simulink model "progetto_sim_controllato"  (R2025b)
settings: Solver=VariableStepAuto  StartTime=0.0  StopTime=1e3  RelTol=1e-3
values from neighbouring files (symbols this model uses):
  d0 = [110 130 100 160]    [backup_id_macchine.mat]    (also in id_macchine.mat)
  dmin = 4    [backup_id_macchine.mat]    (also in id_macchine.mat)
  mDist = [156.727602966 155.419177889 157.307233343 156.111472907]    [backup_id_macchine.mat]    (also in id_macchine.mat = [156.911734511 155.758692096 157.721037406 156.538222818])
  t_cth = 3    [backup_id_macchine.mat]    (also in id_macchine.mat)
  Ts = 2    [backup_id_macchine.mat]    (also in id_macchine.mat)
  umax = 600    [backup_id_macchine.mat]    (also in id_macchine.mat)
  umin = -600    [backup_id_macchine.mat]    (also in id_macchine.mat)
  v0 = [10 12 15 9 10]    [backup_id_macchine.mat]    (also in id_macchine.mat)
  vMedio = [9.99088198605 9.9851530035 9.98261849858 9.98180014012]    [backup_id_macchine.mat]    (also in id_macchine.mat = [10.0026522625 10.0031571294 10.0027874656 10.0025052689])
  x0 = [10 12 15 9 10]    [backup_id_macchine.mat]    (also in id_macchine.mat)
undefined symbols (not defined in the file or in its folder): s2totss, s3totss, s4totss, s5totss
libraries: mpclib x4
settings Model: Creator=david  LastModifiedBy=david

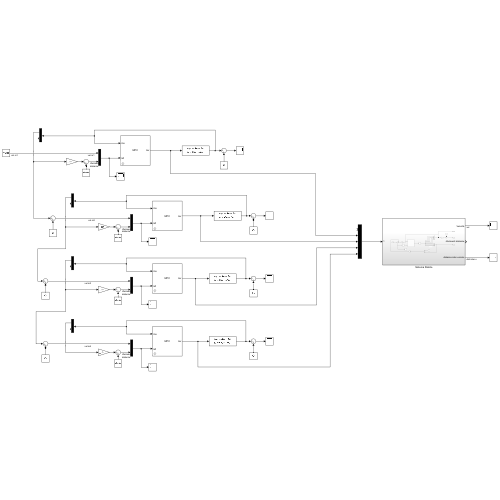
[thumbnail: Simulink's stored preview of the top-level diagram]
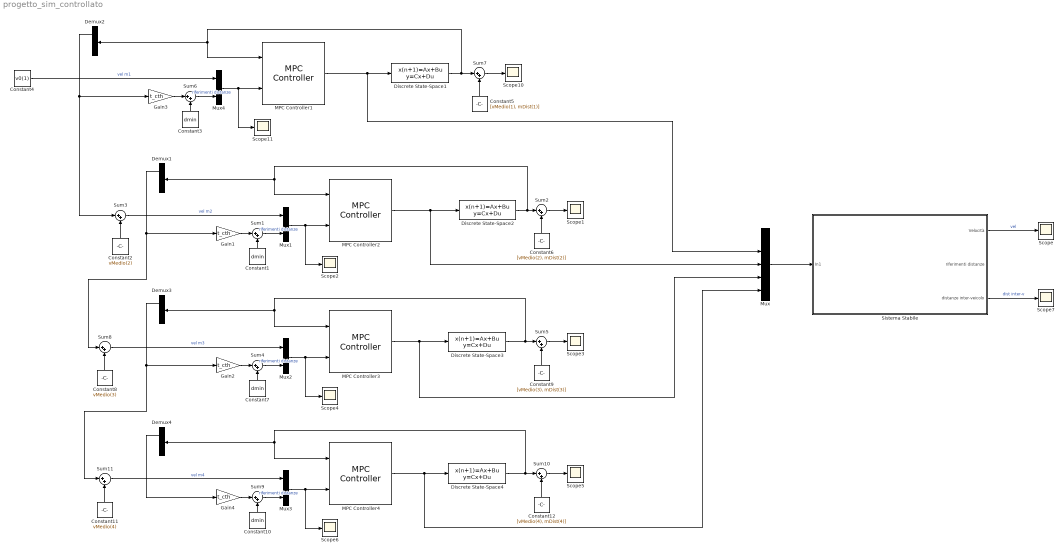
== system progetto_sim_controllato ==
  Constant{1,3,7,10} (4 alike) : Constant  Value=dmin
  Constant11 : Constant  Value=vMedio(4)
  Constant12 : Constant  Value=[vMedio(4), mDist(4)]
  Constant2 : Constant  Value=vMedio(2)
  Constant4 : Constant  Value=v0(1)
  Constant5 : Constant  Value=[vMedio(1), mDist(1)]
  Constant6 : Constant  Value=[vMedio(2), mDist(2)]
  Constant8 : Constant  Value=vMedio(3)
  Constant9 : Constant  Value=[vMedio(3), mDist(3)]
  Demux{1..4} (4 alike) : Demux  Outputs=2
  Discrete State-Space1 : DiscreteStateSpace  A=s2totss.A  B=s2totss.B  C=s2totss.C  D=s2totss.D  SampleTime=Ts
  Discrete State-Space2 : DiscreteStateSpace  A=s3totss.A  B=s3totss.B  C=s3totss.C  D=s3totss.D  SampleTime=Ts
  Discrete State-Space3 : DiscreteStateSpace  A=s4totss.A  B=s4totss.B  C=s4totss.C  D=s4totss.D  SampleTime=Ts
  Discrete State-Space4 : DiscreteStateSpace  A=s5totss.A  B=s5totss.B  C=s5totss.C  D=s5totss.D  SampleTime=Ts
  Gain{1..4} (4 alike) : Gain  Gain=t_cth
  MPC Controller1 : mpclib/MPC Controller  SCDEnableBlockLinearizationSpecification=on  mpcobj=mpcs2  is_multiple=0  enable_value=0  return_u0=off  updateMPCinCallerWorkspace=on  md_inport=off  mv_inport=off  uref_inport=off  return_cost=off  return_mvseq=off  return_qpstatus=off  return_xseq=off  return_state=off  return_ovseq=off  state_inport=off  umin_inport=off  umax_inport=off  ymin_inport=off  ymax_inport=off  cc_inport=off  ywt_inport=off  uwt_inport=off  duwt_inport=off  rhoeps_inport=off  pm_inport=off  MaximumP=10  HorizonChoice=FixedHorizon  n_ts=2  n_p=10  n_mv=1  n_md=0  n_ud=0  n_mo=2  n_uo=0  BlockDataType=double  SampleTimeInherited=off  switch_inport=off
  MPC Controller2 : mpclib/MPC Controller  SCDEnableBlockLinearizationSpecification=on  mpcobj=mpcs3  is_multiple=0  enable_value=0  return_u0=off  updateMPCinCallerWorkspace=on  md_inport=off  mv_inport=off  uref_inport=off  return_cost=off  return_mvseq=off  return_qpstatus=off  return_xseq=off  return_state=off  return_ovseq=off  state_inport=off  umin_inport=off  umax_inport=off  ymin_inport=off  ymax_inport=off  cc_inport=off  ywt_inport=off  uwt_inport=off  duwt_inport=off  rhoeps_inport=off  pm_inport=off  MaximumP=10  HorizonChoice=FixedHorizon  n_ts=2  n_p=10  n_mv=1  n_md=0  n_ud=0  n_mo=2  n_uo=0  BlockDataType=double  SampleTimeInherited=off  switch_inport=off
  MPC Controller3 : mpclib/MPC Controller  SCDEnableBlockLinearizationSpecification=on  mpcobj=mpcs4  is_multiple=0  enable_value=0  return_u0=off  updateMPCinCallerWorkspace=on  md_inport=off  mv_inport=off  uref_inport=off  return_cost=off  return_mvseq=off  return_qpstatus=off  return_xseq=off  return_state=off  return_ovseq=off  state_inport=off  umin_inport=off  umax_inport=off  ymin_inport=off  ymax_inport=off  cc_inport=off  ywt_inport=off  uwt_inport=off  duwt_inport=off  rhoeps_inport=off  pm_inport=off  MaximumP=10  HorizonChoice=FixedHorizon  n_ts=2  n_p=10  n_mv=1  n_md=0  n_ud=0  n_mo=2  n_uo=0  BlockDataType=double  SampleTimeInherited=off  switch_inport=off
  MPC Controller4 : mpclib/MPC Controller  SCDEnableBlockLinearizationSpecification=on  mpcobj=mpcs5  is_multiple=0  enable_value=0  return_u0=off  updateMPCinCallerWorkspace=on  md_inport=off  mv_inport=off  uref_inport=off  return_cost=off  return_mvseq=off  return_qpstatus=off  return_xseq=off  return_state=off  return_ovseq=off  state_inport=off  umin_inport=off  umax_inport=off  ymin_inport=off  ymax_inport=off  cc_inport=off  ywt_inport=off  uwt_inport=off  duwt_inport=off  rhoeps_inport=off  pm_inport=off  MaximumP=10  HorizonChoice=FixedHorizon  n_ts=2  n_p=10  n_mv=1  n_md=0  n_ud=0  n_mo=2  n_uo=0  BlockDataType=double  SampleTimeInherited=off  switch_inport=off
  Mux : Mux  Inputs=5
  Mux{1..4} (4 alike) : Mux  Inputs=2
  Scope{,1..7,10..11} (10 alike) : Scope
      Scope settings: ActiveDisplayYMinimum=7.1891776875022071  ActiveDisplayYMaximum=15.867869145833088  DataLoggingVariableName=ScopeData6
      Scope1 settings: ActiveDisplayYMinimum=10.60470416126369  ActiveDisplayYMaximum=10.628775186898299
      Scope10 settings: ActiveDisplayYMinimum=9.85178753278167  ActiveDisplayYMaximum=10.21313439515283  DataLoggingVariableName=ScopeData21
      Scope11 settings: ActiveDisplayYMinimum=-1  ActiveDisplayYMaximum=1  DataLoggingVariableName=ScopeData22
      Scope2 settings: ActiveDisplayYMinimum=9.99782194789179  ActiveDisplayYMaximum=10.03576388043639
      Scope3 settings: ActiveDisplayYMinimum=9.8157241607277683  ActiveDisplayYMaximum=12.871337364076957  DataLoggingVariableName=ScopeData2
      Scope4 settings: ActiveDisplayYMinimum=9.99782194789179  ActiveDisplayYMaximum=10.03576388043639  DataLoggingVariableName=ScopeData3
      Scope5 settings: ActiveDisplayYMinimum=5.3910159181870654  ActiveDisplayYMaximum=20.171430503682927  DataLoggingVariableName=ScopeData4
      Scope6 settings: ActiveDisplayYMinimum=1.7380163806894  ActiveDisplayYMaximum=24.357852573795405  DataLoggingVariableName=ScopeData5
      Scope7 settings: ActiveDisplayYMinimum=40.1130251052208  ActiveDisplayYMaximum=173.32077498830881  DataLoggingVariableName=ScopeData7
  Sistema Stabile : Subsystem
  Sum{1..11} (11 alike) : Sum  Inputs=|++
  wires:
  Constant5/1 -> Sum7/2
  Sum6/1 -> Mux4/2  "riferimenti distanze"
  Mux4/1 -> Scope11/1, MPC Controller1/2
  Sum7/1 -> Scope10/1
  Constant3/1 -> Sum6/2
  Gain3/1 -> Sum6/1
  MPC Controller1/1 -> Mux/2, Discrete State-Space1/1
  Discrete State-Space1/1 -> Sum7/1, MPC Controller1/1, Demux2/1
  Gain1/1 -> Sum1/1
  MPC Controller2/1 -> Mux/3, Discrete State-Space2/1
  Discrete State-Space2/1 -> MPC Controller2/1, Demux1/1, Sum2/1
  Sum1/1 -> Mux1/2  "riferimenti distanze"
  Mux1/1 -> Scope2/1, MPC Controller2/2
  Demux1/1 -> Sum8/1, Gain1/1
  Constant1/1 -> Sum1/2
  Sum2/1 -> Scope1/1
  Constant6/1 -> Sum2/2
  Sum3/1 -> Mux1/1  "vel m2"
  Constant2/1 -> Sum3/2
  Demux3/1 -> Sum11/1, Gain2/1
  Constant7/1 -> Sum4/2
  Sum5/1 -> Scope3/1
  Constant9/1 -> Sum5/2
  Mux2/1 -> Scope4/1, MPC Controller3/2
  Discrete State-Space3/1 -> Sum5/1, MPC Controller3/1, Demux3/1
  Gain2/1 -> Sum4/1
  MPC Controller3/1 -> Mux/4, Discrete State-Space3/1
  Sum4/1 -> Mux2/2  "riferimenti distanze"
  Constant8/1 -> Sum8/2
  Sum8/1 -> Mux2/1  "vel m3"
  Demux2/1 -> Sum3/1, Gain3/1
  Sum11/1 -> Mux3/1  "vel m4"
  Constant11/1 -> Sum11/2
  Sum9/1 -> Mux3/2  "riferimenti distanze"
  MPC Controller4/1 -> Mux/5, Discrete State-Space4/1
  Gain4/1 -> Sum9/1
  Discrete State-Space4/1 -> Sum10/1, MPC Controller4/1, Demux4/1
  Mux3/1 -> Scope6/1, MPC Controller4/2
  Constant10/1 -> Sum9/2
  Sum10/1 -> Scope5/1
  Demux4/1 -> Gain4/1
  Constant12/1 -> Sum10/2
  Constant4/1 -> Mux4/1  "vel m1"
  Mux/1 -> Sistema Stabile/1(In1)
  Sistema Stabile/1(Velocità) -> Scope/1  "vel"
  Sistema Stabile/3(distanze inter-veicolo) -> Scope7/1  "dist inter-v"

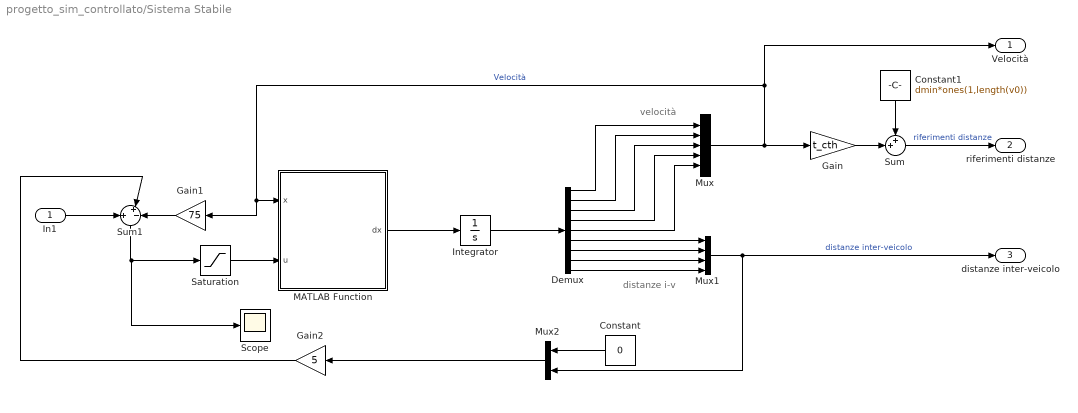
== system progetto_sim_controllato/Sistema Stabile ==
  note: distanze i-v
  note: velocità
  In1 : Inport
  Constant : Constant  Value=0
  Constant1 : Constant  Value=dmin*ones(1,length(v0))
  Demux : Demux  Outputs=9
  Gain : Gain  Gain=t_cth
  Gain1 : Gain  Gain=75
  Gain2 : Gain  Gain=5
  Integrator : Integrator  InitialCondition=[x0,d0]
  MATLAB Function : MATLAB Function  TreatAsAtomicUnit=on
  Mux : Mux  Inputs=5
  Mux1 : Mux
  Mux2 : Mux  Inputs=2
  Saturation : Saturate  UpperLimit=umax  LowerLimit=umin
  Scope : Scope
      settings: ActiveDisplayYMinimum=-870.07079552701  ActiveDisplayYMaximum=313.69351903872894  DataLoggingVariableName=ScopeData18
  Sum : Sum  Inputs=++|
  Sum1 : Sum  Inputs=+|+-
  Velocità : Outport
  riferimenti distanze : Outport  Port=2
  distanze inter-veicolo : Outport  Port=3
  wires:
  Mux/1 -> Gain1/1, MATLAB Function/1(x), Velocità/1, Gain/1  "Velocità"
  Demux/6 -> Mux1/1
  Saturation/1 -> MATLAB Function/2(u)
  Demux/4 -> Mux/4
  Integrator/1 -> Demux/1
  Demux/1 -> Mux/1
  Demux/8 -> Mux1/3
  Demux/3 -> Mux/3
  MATLAB Function/1(dx) -> Integrator/1
  Demux/2 -> Mux/2
  Demux/7 -> Mux1/2
  Demux/5 -> Mux/5
  Gain/1 -> Sum/2
  Constant1/1 -> Sum/1
  Sum1/1 -> Scope/1, Saturation/1
  Demux/9 -> Mux1/4
  Sum/1 -> riferimenti distanze/1  "riferimenti distanze"
  Mux1/1 -> Mux2/2, distanze inter-veicolo/1  "distanze inter-veicolo"
  In1/1 -> Sum1/1
  Constant/1 -> Mux2/1
  Mux2/1 -> Gain2/1
  Gain1/1 -> Sum1/3
  Gain2/1 -> Sum1/2

== matlab function progetto_sim_controllato/Sistema Stabile/MATLAB Function ==
  data: x input; u input size=[1 5]; dx output size=[1 9]
function dx = sistemaVeicoli5(x, u)
% sistemaVeicoli5 - Modello dinamico 5 veicoli platooning
%
% Inputs:
%   t     - tempo (per integratori)
%   x     - stato: [v1, v2, v3, v4, v5, d2, d3, d4, d5]
%   u     - forze trazione [u1, u2, u3, u4, u5]
%
% Outputs:
%   dx    - derivata degli stati

m = [790 820 760 860 800];

rho = 1.22;        % Densità aria kg/m^3
caA = 0.88;        % Coeff Aerodinamico * superficie
cr = 0.01;         % Resistenza rotolamento stimata
gr = 9.81;         % Gravità

v = x(1:5);        % velocità
    
dv = zeros(1,5);
dd = zeros(1,4);

for i = 2:5
    FL = 0.5 * rho * caA * v(i)^2 + cr * m(i) * gr;
    dv(i) = (u(i) - FL) / m(i);

    dd(i-1) = v(i-1) - v(i);
end

dx = [dv'; dd']';

end
